simulink library "drone"  (R2022a)
settings: Solver=VariableStepAuto  StartTime=0.0  StopTime=10.0  RelTol=1e-3
settings Model: Creator=JadKHaddad  LastModifiedBy=JadKHaddad

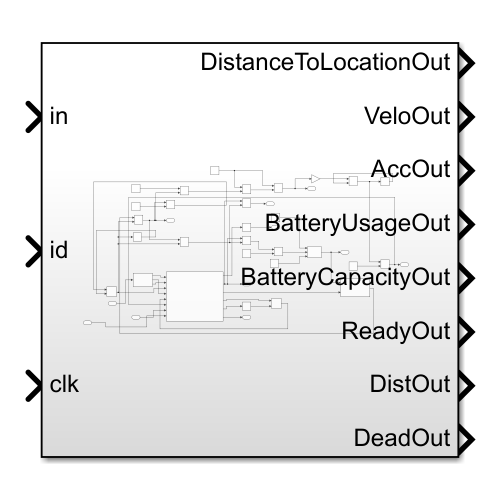
[thumbnail: Simulink's stored preview of the top-level diagram]
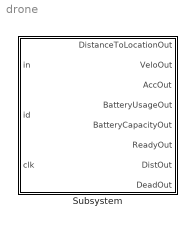
== system drone ==
  Subsystem : Subsystem

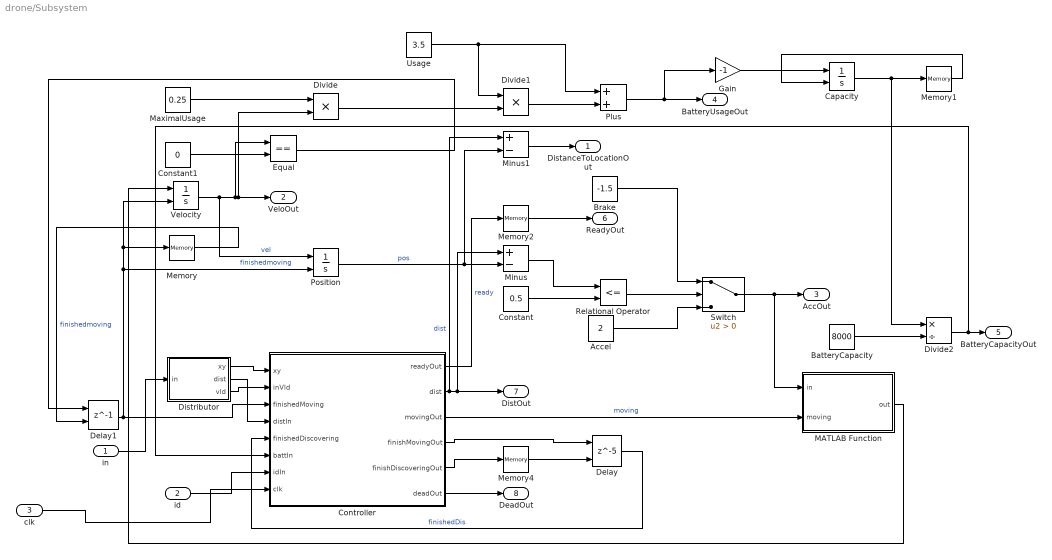
== system drone/Subsystem ==
  in : Inport
  id : Inport  Port=2
  clk : Inport  Port=3
  Accel : Constant  Value=2
  BatteryCapacity : Constant  Value=8000
  Brake : Constant  Value=-1.5
  Capacity : Integrator  ExternalReset=rising  InitialCondition=8000  LowerSaturationLimit=0
  Constant : Constant  Value=0.5
  Constant1 : Constant  Value=0
  Controller : MATLAB Function  TreatAsAtomicUnit=on
  Delay : Delay  DelayLength=5  InitialCondition=0  ExternalReset=Rising
      settings: InputPortMap=u0,r5
  Delay1 : Delay  DelayLength=1  ExternalReset=Rising
      settings: InputPortMap=u0,r5
  Distributor : MATLAB Function  TreatAsAtomicUnit=on
  Divide : Product  Inputs=**  RndMeth=Round
  Divide1 : Product  Inputs=**
  Divide2 : Product  Inputs=*/
  Equal : RelationalOperator  Operator===  OutDataTypeStr=boolean  RndMeth=Simplest  InputSameDT=off
  Gain : Gain  Gain=-1
  MATLAB Function : MATLAB Function  TreatAsAtomicUnit=on
  MaximalUsage : Constant  Value=0.25
  Memory : Memory  InheritSampleTime=on
  Memory1 : Memory
  Memory2 : Memory
  Memory4 : Memory
  Minus : Sum  Inputs=+-
  Minus1 : Sum  Inputs=+-
  Plus : Sum
  Position : Integrator  ExternalReset=rising
  Relational Operator : RelationalOperator  Operator=<=  OutDataTypeStr=boolean  RndMeth=Simplest  InputSameDT=off
  Switch : Switch  Criteria=u2 > Threshold  SaturateOnIntegerOverflow=off  InputSameDT=off
  Usage : Constant  Value=3.5
  Velocity : Integrator  ExternalReset=rising  LimitOutput=on  UpperSaturationLimit=1  LowerSaturationLimit=0
  DistanceToLocationOut : Outport
  VeloOut : Outport  Port=2
  AccOut : Outport  Port=3
  BatteryUsageOut : Outport  Port=4
  BatteryCapacityOut : Outport  Port=5
  ReadyOut : Outport  Port=6
  DistOut : Outport  Port=7
  DeadOut : Outport  Port=8
  wires:
  Gain/1 -> Capacity/1
  Controller/6(deadOut) -> DeadOut/1
  Divide/1 -> Divide1/2
  id/1 -> Controller/7(idIn)
  Minus/1 -> Relational Operator/1
  Accel/1 -> Switch/3
  Memory/1 -> Delay1/2  "finishedmoving"
  Minus1/1 -> DistanceToLocationOut/1
  Capacity/1 -> Memory1/1, Divide2/1
  Distributor/3(vld) -> Controller/2(inVld)
  Distributor/1(xy) -> Controller/1(xy)
  Memory1/1 -> Capacity/2
  Constant/1 -> Relational Operator/2
  Distributor/2(dist) -> Controller/4(distIn)
  Memory4/1 -> Delay/2
  Relational Operator/1 -> Switch/2
  BatteryCapacity/1 -> Divide2/2
  Divide1/1 -> Plus/2
  Plus/1 -> Gain/1, BatteryUsageOut/1
  Brake/1 -> Switch/1
  Constant1/1 -> Equal/2
  Position/1 -> Minus1/2, Minus/2  "pos"
  Memory2/1 -> ReadyOut/1
  MATLAB Function/1(out) -> Velocity/1
  Equal/1 -> Delay1/1
  Controller/5(finishDiscoveringOut) -> Memory4/1
  Controller/3(movingOut) -> MATLAB Function/2(moving)  "moving"
  Delay1/1 -> Velocity/2, Memory/1, Position/2, Controller/3(finishedMoving)  "finishedmoving"
  Divide2/1 -> BatteryCapacityOut/1, Controller/6(battIn)
  Controller/1(readyOut) -> Memory2/1  "ready"
  Controller/4(finishMovingOut) -> Delay/1
  in/1 -> Distributor/1(in)
  Switch/1 -> MATLAB Function/1(in), AccOut/1
  MaximalUsage/1 -> Divide/1
  Delay/1 -> Controller/5(finishedDiscovering)  "finishedDis"
  Usage/1 -> Plus/1, Divide1/1
  Velocity/1 -> Divide/2, VeloOut/1, Equal/1, Position/1  "vel"
  Controller/2(dist) -> DistOut/1, Minus/1, Minus1/1  "dist"
  clk/1 -> Controller/8(clk)

== matlab function drone/Subsystem/Distributor ==
  data: in input; xy output; dist output; vld output
function [xy, dist, vld] = fcn(in)
    %distributes an input signal to multiple output signals
    xy = [-1 -1];
    dist = -1;
    vld = 0;
    
    xy = [in(1) in(2)];
    dist = in(3);
    vld = in(4);
end

== matlab function drone/Subsystem/Controller ==
  settings: updateMethod=DISCRETE
  data: xy input; readyOut output; inVld input; finishedMoving input; dist output; distIn input; finishedDiscovering input; movingOut output; finishMovingOut output; finishDiscoveringOut output; battIn input; idIn input; deadOut output; clk input
function [readyOut, dist, movingOut, finishMovingOut, finishDiscoveringOut, deadOut] = fcn(xy, inVld, finishedMoving, distIn, finishedDiscovering, battIn, idIn, clk)
    persistent distance
    persistent ready
    persistent moving
    persistent ignoreMoving
    persistent ignoreDiscovering
    persistent discovering
    persistent terminate
    persistent dead
    
    %init persistent values
    if isempty(dead)
        dead = 0;
    end
    if isempty(terminate)
        terminate = 0;
    end
    if isempty(ignoreMoving)
        ignoreMoving = 1;
    end
    if isempty(ignoreDiscovering)
        ignoreDiscovering = 1;
    end
    if isempty(ready)
        ready = 1;
    end
    
    if isempty(moving)
        moving = 0;
    end
    
    if isempty(discovering)
        discovering = 0;
    end
    if isempty(distance)
        distance = -1;
    end
    
    finishMovingOut = 0;
    finishDiscoveringOut = 0;
    
    %if the drone finished moving it should start discovering
    if finishedMoving == 1 && ignoreMoving == 0
        if moving == 1
            moving = 0;
            finishMovingOut = 1;
            discovering = 1;
            ignoreMoving = 1;
            ignoreDiscovering = 0;
        end
    end
    
    %if the drone finished discovering it should be ready again
    if finishedDiscovering == 1 && ignoreDiscovering == 0
        if discovering == 1
            ignoreDiscovering = 1;
            discovering = 0;
            finishDiscoveringOut = 1;
        end
    end
    
    %a new position has been given - drone should move to the given
    %position and start discovering
    if inVld == 1 && ready == 1
        ready = 0;
        distance = distIn;
        moving = 1;
        ignoreMoving = 0;
        discovering = 0;
        if xy(1) == -2
            terminate = 1;
        end
    end
    
    %a drone can't receive new positions while moving or discovering
    if discovering == 1 || moving == 1
        ready = 0;
    end
    
    %a drone is ready if it is not moving or discovering
    if discovering == 0 && moving == 0
        ready = 1;
    end
    
    if discovering == 1 && moving == 0 && terminate == 1
        ready = 1;
    end
    
    %if battery dies, the drone is lost
    if battIn <= 0
       discovering = 0;
       moving = 0;
       ready = 0;
       if dead == 0
           fprintf("[%d]: Drone [%d] died\n",int32(clk), int8(idIn));
       end
       dead = 1;
    end
    
    dist = distance;
    movingOut = moving;
    readyOut = ready;
    deadOut = dead;
end

== matlab function drone/Subsystem/MATLAB Function ==
  data: in input; out output; moving input
function out = fcn(in, moving)
    %prevents drone from moving if it is not supposed to move
    out = 0;
    if moving == 1
        out = in;
    end
end
